simulink model "proj2"  (Simulink 7.7)
settings: Solver=ode45  StartTime=0.0  StopTime=80  RelTol=1e-3
values from neighbouring files (symbols this model uses):
  B = -inv(A)*C    [proj.m]
  Cir = fill(x1,y1,'r')    [proj.m]
  D = -inv(A)*G    [proj.m]
  K = lqr(T,Q,Qr,R)    [proj.m]
  Q = [0;0;Q]    [proj.m]
  Squ = fill(x2,y2,'b')    [proj.m]
undefined symbols (not defined in the file or in its folder): sigbuilder_block, simule
libraries: simulink x2
settings Model: Creator=Owner  LastModifiedBy=Owner
settings OptimizationCC: InlineInvariantSignals=on  InitFltsAndDblsToZero=on
settings DebuggingCC: SaveWithParameterizedLinksMsg=none  SignalResolutionControl=TryResolveAllWithWarning  MultiTaskDSMMsg=warning  MultiTaskCondExecSysMsg=none  StrictBusMsg=None
settings RTWCC: IncludeERTFirstTime=on
settings GRTTargetCC: TargetFcnLib=ansi_tfl_tmw.mat

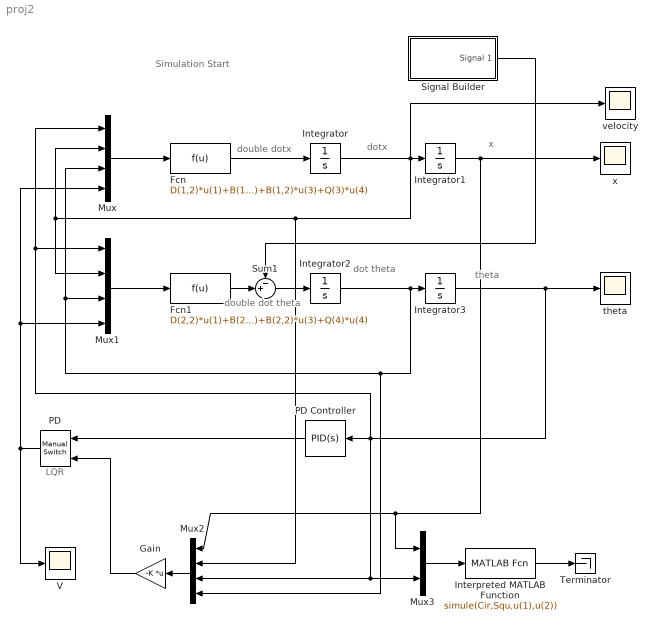
== system proj2 ==
  note: x
  note: dotx
  note: double dotx
  note: double dot
      | theta
  note: dot theta
  note: theta
  note: Simulation Start
  note: LQR
  Fcn : Fcn  Expr=D(1,2)*u(1)+B(1,1)*u(2)+B(1,2)*u(3)+Q(3)*u(4)
  Fcn1 : Fcn  Expr=D(2,2)*u(1)+B(2,1)*u(2)+B(2,2)*u(3)+Q(4)*u(4)
  Gain : Gain  Gain=-K  Multiplication=Matrix(K*u)
  Integrator : Integrator
  Integrator1 : Integrator
  Integrator2 : Integrator
  Integrator3 : Integrator  InitialCondition=0.11
  Interpreted MATLAB Function : MATLABFcn  MATLABFcn=simule(Cir,Squ,u(1),u(2))
  Mux : Mux
  Mux1 : Mux
  Mux2 : Mux
  Mux3 : Mux  Inputs=2
  PD : simulink/Signal Routing/Manual Switch  SystemSampleTime=-1  sw=0  action=0  varsize=off
  PD Controller : simulink/Continuous/PID Controller  SystemSampleTime=-1  Controller=PID  TimeDomain=Continuous-time  SampleTime=1  IntegratorMethod=Forward Euler  FilterMethod=Forward Euler  Form=Parallel  P=-K(2)  I=0  D=-K(4)  N=100  InitialConditionSource=internal  InitialConditionForIntegrator=0  InitialConditionForFilter=0  ExternalReset=none  LimitOutput=on  UpperSaturationLimit=12  LowerSaturationLimit=-12  LinearizeAsGain=off  AntiWindupMode=none  Kb=1  TrackingMode=off  Kt=1  PParamMin=[]  PParamMax=[]  IParamMin=[]  IParamMax=[]  DParamMin=[]  DParamMax=[]  NParamMin=[]  NParamMax=[]  KbParamMin=[]  KbParamMax=[]  KtParamMin=[]  KtParamMax=[]  POutMin=[]  POutMax=[]  IOutMin=[]  IOutMax=[]  DOutMin=[]  DOutMax=[]  NOutMin=[]  NOutMax=[]  KbOutMin=[]  KbOutMax=[]  KtOutMin=[]  KtOutMax=[]  IntegratorOutMin=[]  IntegratorOutMax=[]  FilterOutMin=[]  FilterOutMax=[]  SumOutMin=[]  SumOutMax=[]  SumI1OutMin=[]  SumI1OutMax=[]  SumI2OutMin=[]  SumI2OutMax=[]  SumI3OutMin=[]  SumI3OutMax=[]  SumDOutMin=[]  SumDOutMax=[]  SaturationOutMin=[]  SaturationOutMax=[]  IntegratorContinuousStateAttributes=''  IntegratorStateMustResolveToSignalObject=off  IntegratorRTWStateStorageClass=Auto  FilterContinuousStateAttributes=''  FilterStateMustResolveToSignalObject=off  FilterRTWStateStorageClass=Auto
  Signal Builder : Subsystem  Tag=STV Subsys  LoadFcn=sigbuilder_block('load',[172.5 51.75 304.5 229.5 ]);  StartFcn=sigbuilder_block('start');  StopFcn=sigbuilder_block('stop');  ClipboardFcn=sigbuilder_block('clipboard');  mask(Sigbuilder block){}
      mask help: Create and generate interchangeable groups of signals whose waveforms are piecewise linear.
      mask init:
      | if ~strcmp(get_param(bdroot(gcbh),'SimulationStatus'),'stopped') tuvar = sigbuilder_block('maskInit'); end
      settings: CopyFcn=sigbuilder_block('copy');  DeleteFcn=sigbuilder_block('delete');  ModelCloseFcn=sigbuilder_block('modelClose');  PreSaveFcn=sigbuilder_block('preSave');  NameChangeFcn=sigbuilder_block('namechange');  OpenFcn=sigbuilder_block('open',[140.25 195 550.5 399.75 ]);  CloseFcn=sigbuilder_block('close');
      mask Display: plot(0, 0, 100, 100,[2, 2, 32, 32, 2], [68, 8, 8, 68, 68],[32, 2], [38, 38], [32, 19, 2],[53, 60, 44], [32, 17, 17, 2],[16, 16, 31, 31]);txt = getActiveGroup(gcbh);text(2, 100, txt,'verticalAlignment', 'top');
  Sum1 : Sum  Inputs=-+|
  Terminator : Terminator
  V : Scope
      settings: YMin=-12  YMax=4  SaveName=ScopeData2
  theta : Scope
      settings: YMin=-0.2  YMax=0.45
  velocity : Scope
      settings: YMin=-0.45  YMax=0.25  SaveName=ScopeData3
  x : Scope
      settings: YMin=-2  YMax=0.25
  wires:
  Integrator/1 -> Mux/2, Mux1/2, Mux2/2, Integrator1/1, velocity/1
  Integrator1/1 -> x/1, Mux3/1, Mux2/1
  Fcn/1 -> Integrator/1
  Mux/1 -> Fcn/1
  Integrator2/1 -> Integrator3/1, Mux1/3, Mux/3, Mux2/4
  Mux1/1 -> Fcn1/1
  PD Controller/1 -> PD/1
  Mux3/1 -> Interpreted MATLAB Function/1
  Interpreted MATLAB Function/1 -> Terminator/1
  Integrator3/1 -> theta/1, PD Controller/1, Mux1/1, Mux/1, Mux3/2, Mux2/3
  Gain/1 -> PD/2
  Mux2/1 -> Gain/1
  PD/1 -> Mux1/4, Mux/4, V/1
  Fcn1/1 -> Sum1/2
  Sum1/1 -> Integrator2/1
  Signal Builder/1(Signal 1) -> Sum1/1

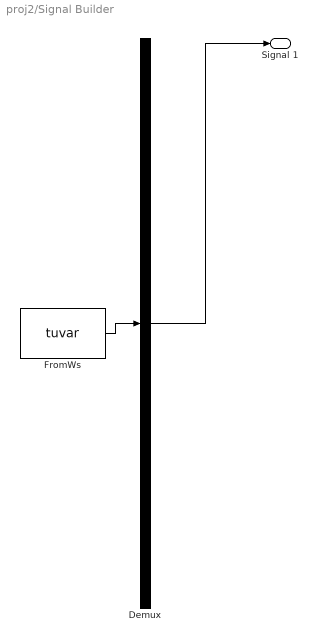
== system proj2/Signal Builder ==
  Demux : Demux  Tag=STV Demux  Outputs=1
  FromWs : FromWorkspace  Tag=STV FromWs  VariableName=tuvar  SampleTime=0  SigBuilderData=DataTag0  VnvData=DataTag1
      SigBuilderData=|
      | common.afterFinalStr = 'Extrapolate'
      | common.sampleTime = 0
      | dataSet.timeRange = [0 10]
      | dataSet.name = 'Group 1'
      | sbobj.Groups.Name = 'Group 1'
      | sbobj.Groups.Signals.Name = 'Signal 1'
      | sbobj.Groups.Signals.XData = [0 0.35 2.05 3.78 4.84 5.66 6.64 8.1 9.04 10]
      | sbobj.Groups.Signals.YData = [0.02 0.02 2.45 1.45 0.02 0.02 -3.3 -2.55 0.02 0.02]
  Signal 1 : Outport  Tag=STV Outport
  wires:
  Demux/1 -> Signal 1/1
  FromWs/1 -> Demux/1
